simulink model "duocopter simulink model"  (R2020b)
settings: Solver=ode45  StartTime=0.0  StopTime=60  MaxStep=0.1  RelTol=1e-3
model workspace (MAT data in the model file):
  center_rotor_distance = 0.1
  mass_drone = 0.661
  moment_inertia_drone = [0.0019  0  0.0001; 0  0.004  0; 0.0001  0  0.0021]
  thrust_per_motor = 8.6328
libraries: simulink x6, pid_lib x3, shared6dof x1, robotcorelib x1, simulink_extras x1, sharedtransform x1, uavutilslib x1
settings Model: PacingRate=3  Creator=thega  LastModifiedBy=thega
settings DataIOCC: ReturnWorkspaceOutputsName=tp49ac784a_13d7_45a6_aa80_7f0641734b4f

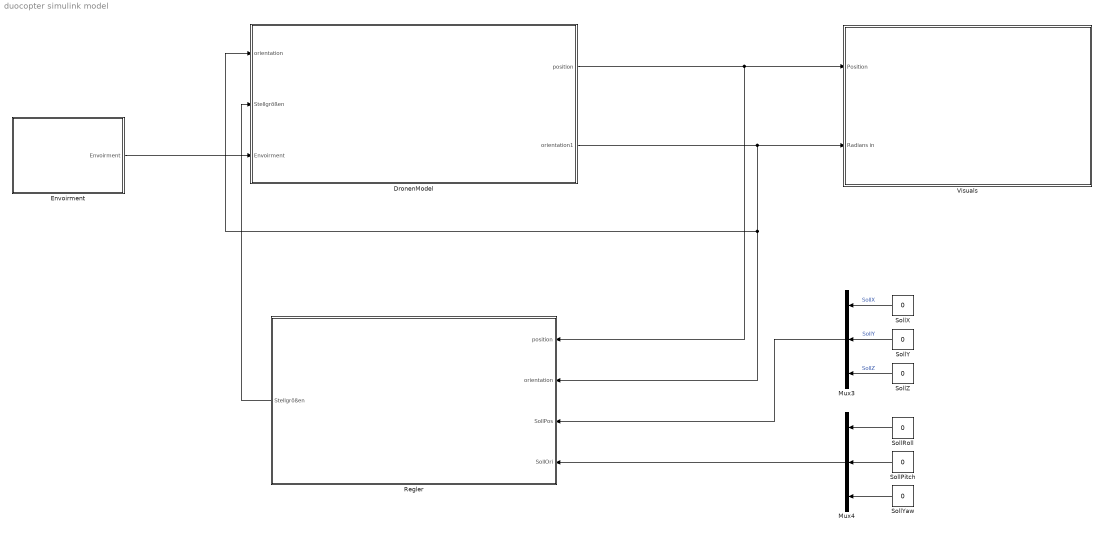
== system duocopter simulink model ==
  DronenModel : Subsystem
  Envoirment : Subsystem
  Mux3 : Mux  Inputs=3
  Mux4 : Mux  Inputs=3
  Regler : Subsystem
  SollPitch : Constant  Value=0
  SollRoll : Constant  Value=0
  SollX : Constant  Value=0
  SollY : Constant  Value=0
  SollYaw : Constant  Value=0
  SollZ : Constant  Value=0
  Visuals : Subsystem
  wires:
  SollX/1 -> Mux3/1  "SollX"
  SollY/1 -> Mux3/2  "SollY"
  SollZ/1 -> Mux3/3  "SollZ"
  SollYaw/1 -> Mux4/3
  SollPitch/1 -> Mux4/2
  SollRoll/1 -> Mux4/1
  Mux3/1 -> Regler/3(SollPos)
  Mux4/1 -> Regler/4(SollOri)
  DronenModel/1(position) -> Regler/1(position), Visuals/1(Position)
  DronenModel/2(orientation1) -> Visuals/2(Radians in), DronenModel/1(orientation), Regler/2(orientation)
  Regler/1(Stellgrößen) -> DronenModel/2(Stellgrößen)
  Envoirment/1(Envoirment) -> DronenModel/3(Envoirment)

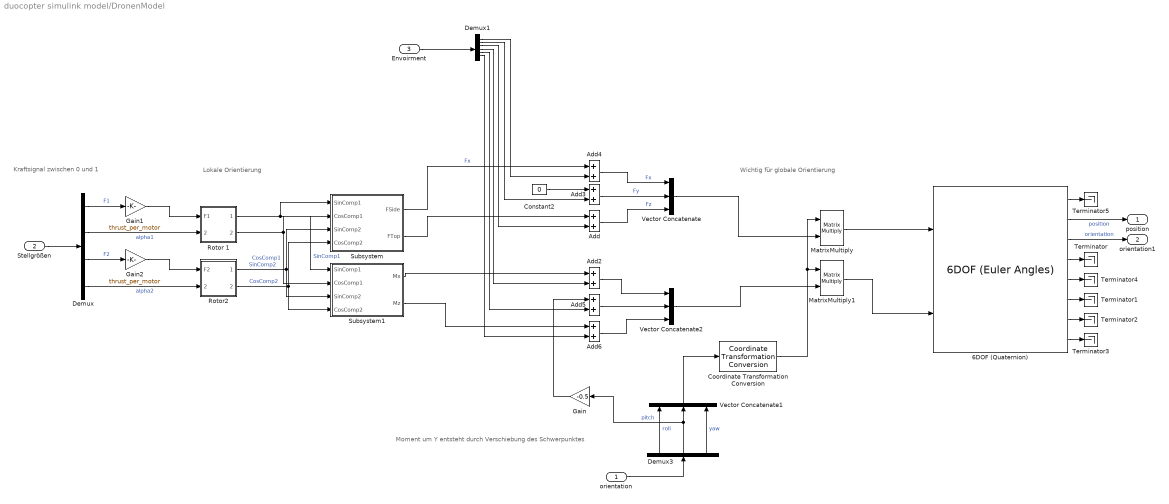
== system duocopter simulink model/DronenModel ==
  note: Kraftsignal zwischen 0 und 1
  note: Moment um Y entsteht durch Verschiebung des Schwerpunktes
  note: Lokale Orientierung
  note: Wichtig für globale Orientierung
  orientation : Inport
  Stellgrößen : Inport  Port=2
  Envoirment : Inport  Port=3
  6DOF (Quaternion) : shared6dof/6DOF (Euler Angles)  units=Metric (MKS)  mtype=Fixed  rep=Quaternion  xme_0=[0 0 0]  Vm_0=[0 0 0]  eul_0=[0 0 0]  pm_0=[0 0 0]  mass_0=mass_drone  mass_e=0.5  mass_f=2.0  inertia=moment_inertia_drone  inertia_e=eye(3)  inertia_f=2*eye(3)  k_quat=1.0  vre_flag=on  abi_flag=off  aMode=0  xme_statename=''  Vm_statename=''  eul_statename=''  quat_statename=''  pm_statename=''  mass_statename=''
      settings: SourceProductBaseCode=AE,PW,MT,UV,VE,VP
  Add{,2..6} (6 alike) : Sum
  Constant2 : Constant  Value=0
  Coordinate Transformation Conversion : robotcorelib/Coordinate Transformation Conversion  InputRepresentation=Euler Angles  InputEulerSequence=XYZ  ShowTrVecInputPort=on  OutputRepresentation=Rotation Matrix  OutputEulerSequence=ZYX  ShowTrVecOutputPort=on  SimulateUsing=Interpreted execution
      settings: SourceProductBaseCode=NV,RO,RR,UV
  Demux : Demux
  Demux1 : Demux  Outputs=6
  Demux3 : Demux  Outputs=3
  Gain : Gain  Gain=-0.5
  Gain1 : Gain  Gain=thrust_per_motor
  Gain2 : Gain  Gain=thrust_per_motor
  MatrixMultiply : Product  Multiplication=Matrix(*)
  MatrixMultiply1 : Product  Multiplication=Matrix(*)
  Rotor 1 : Subsystem
  Rotor2 : Subsystem
  Subsystem : Subsystem
  Subsystem1 : Subsystem
  Terminator{,1..5} (6 alike) : Terminator
  Vector Concatenate : Concatenate  NumInputs=3
  Vector Concatenate1 : Concatenate  NumInputs=3
  Vector Concatenate2 : Concatenate  NumInputs=3
  position : Outport
  orientation1 : Outport  Port=2
  wires:
  Add/1 -> Vector Concatenate/3  "Fz"
  6DOF (Quaternion)/8 -> Terminator3/1
  Demux3/3 -> Vector Concatenate1/3  "yaw"
  6DOF (Quaternion)/3 -> orientation1/1  "orientation"
  Rotor 1/2(Out2) -> Subsystem1/2(CosComp1), Subsystem/2(CosComp1)  "CosComp1"
  Rotor 1/1(Out1) -> Subsystem/1(SinComp1), Subsystem1/1(SinComp1)  "SinComp1"
  Subsystem/1(FSide) -> Add4/1  "Fx"
  Demux/1 -> Gain1/1  "F1"
  Subsystem1/1(Mx) -> Add2/1
  orientation/1 -> Demux3/1
  Rotor2/2(Out2) -> Subsystem1/4(CosComp2), Subsystem/4(CosComp2)  "CosComp2"
  Subsystem/2(FTop) -> Add/1
  Demux/2 -> Rotor 1/2(alpha1)  "alpha1"
  Demux3/1 -> Vector Concatenate1/1  "roll"
  Demux/4 -> Rotor2/2(alpha2)  "alpha2"
  6DOF (Quaternion)/7 -> Terminator2/1
  Rotor2/1(Out1) -> Subsystem1/3(SinComp2), Subsystem/3(SinComp2)  "SinComp2"
  Demux3/2 -> Gain/1, Vector Concatenate1/2  "pitch"
  6DOF (Quaternion)/2 -> position/1  "position"
  MatrixMultiply/1 -> 6DOF (Quaternion)/1
  6DOF (Quaternion)/4 -> Terminator/1
  Demux/3 -> Gain2/1  "F2"
  6DOF (Quaternion)/6 -> Terminator1/1
  6DOF (Quaternion)/1 -> Terminator5/1
  6DOF (Quaternion)/5 -> Terminator4/1
  Add3/1 -> Vector Concatenate/2  "Fy"
  Vector Concatenate/1 -> MatrixMultiply/2
  Vector Concatenate1/1 -> Coordinate Transformation Conversion/1
  Coordinate Transformation Conversion/1 -> MatrixMultiply/1, MatrixMultiply1/1
  Add2/1 -> Vector Concatenate2/1
  Add5/1 -> Vector Concatenate2/2
  Subsystem1/2(Mz) -> Add6/1
  Vector Concatenate2/1 -> MatrixMultiply1/2
  MatrixMultiply1/1 -> 6DOF (Quaternion)/2
  Add4/1 -> Vector Concatenate/1  "Fx"
  Demux1/2 -> Add3/2
  Demux1/1 -> Add4/2
  Demux1/3 -> Add/2
  Envoirment/1 -> Demux1/1
  Gain/1 -> Add5/1
  Add6/1 -> Vector Concatenate2/3
  Demux1/4 -> Add2/2
  Demux1/5 -> Add5/2
  Demux1/6 -> Add6/2
  Stellgrößen/1 -> Demux/1
  Constant2/1 -> Add3/1
  Gain1/1 -> Rotor 1/1(F1)
  Gain2/1 -> Rotor2/1(F2)

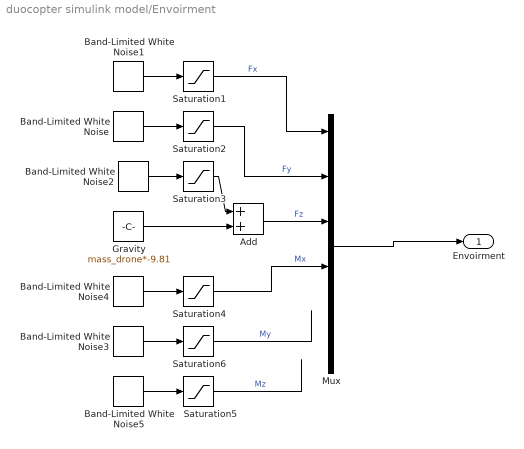
== system duocopter simulink model/Envoirment ==
  Add : Sum
  Band-Limited White Noise : simulink/Sources/Band-Limited White Noise  Cov=[0.1]  Ts=0.1  seed=[41]
  Band-Limited White Noise1 : simulink/Sources/Band-Limited White Noise  Cov=[0.1]  Ts=0.1  seed=[23222241]
  Band-Limited White Noise2 : simulink/Sources/Band-Limited White Noise  Cov=[0.1]  Ts=0.1  seed=[23341]
  Band-Limited White Noise3 : simulink/Sources/Band-Limited White Noise  Cov=[0.1]  Ts=0.1  seed=[67821]
  Band-Limited White Noise4 : simulink/Sources/Band-Limited White Noise  Cov=[0.001]  Ts=0.1  seed=[23678]
  Band-Limited White Noise5 : simulink/Sources/Band-Limited White Noise  Cov=[0.1]  Ts=0.1  seed=[2330]
  Gravity : Constant  Value=mass_drone*-9.81
  Mux : Mux  Inputs=6
  Saturation{1..3,5..6} (5 alike) : Saturate  UpperLimit=0.1  LowerLimit=-.1
  Saturation4 : Saturate  UpperLimit=0.001  LowerLimit=-.0001
  Envoirment : Outport
  wires:
  Mux/1 -> Envoirment/1
  Add/1 -> Mux/3  "Fz"
  Gravity/1 -> Add/2
  Band-Limited White Noise2/1 -> Saturation3/1
  Band-Limited White Noise/1 -> Saturation2/1
  Band-Limited White Noise1/1 -> Saturation1/1
  Band-Limited White Noise4/1 -> Saturation4/1
  Band-Limited White Noise3/1 -> Saturation6/1
  Band-Limited White Noise5/1 -> Saturation5/1
  Saturation1/1 -> Mux/1  "Fx"
  Saturation2/1 -> Mux/2  "Fy"
  Saturation3/1 -> Add/1
  Saturation4/1 -> Mux/4  "Mx"
  Saturation6/1 -> ?  "My"
  Saturation5/1 -> ?  "Mz"

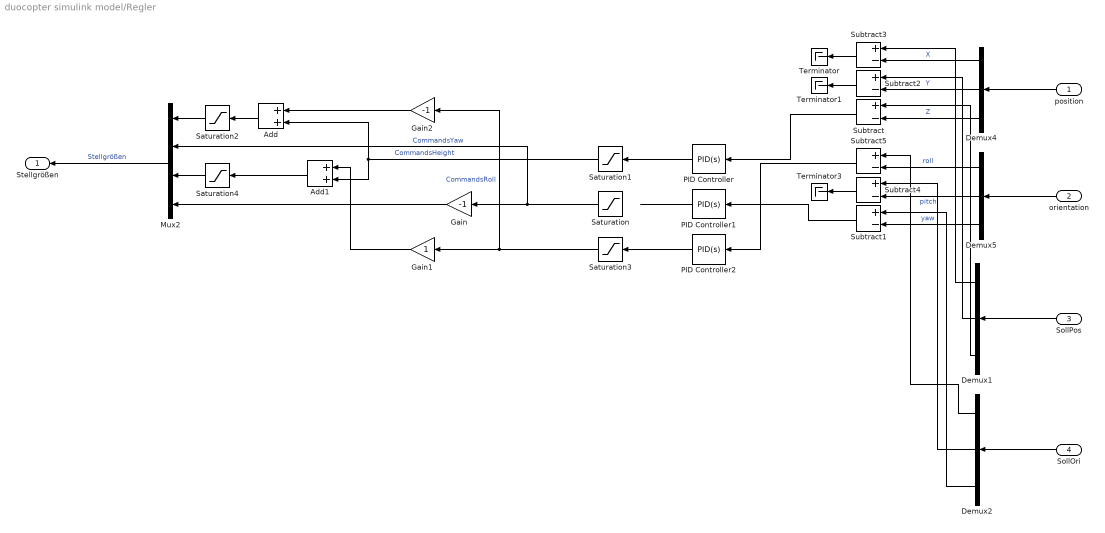
== system duocopter simulink model/Regler ==
  position : Inport
  orientation : Inport  Port=2
  SollPos : Inport  Port=3
  SollOri : Inport  Port=4
  Add : Sum
  Add1 : Sum
  Demux{1..2,4..5} (4 alike) : Demux  Outputs=3
  Gain : Gain  Gain=-1
  Gain1 : Gain
  Gain2 : Gain  Gain=-1
  Mux2 : Mux
  PID Controller : pid_lib/PID Controller  Controller=PID  Form=Parallel  TimeDomain=Continuous-time  UseExternalTs=off  SampleTime=-1  IntegratorMethod=Forward Euler  FilterMethod=Forward Euler  ControllerParametersSource=internal  P=0.0188303154649847  I=0.00247755067319415  D=0.0356353845754746  UseFilter=on  N=114.28279760416  TunerSelectOption=Transfer Function Based (PID Tuner App)  InitialConditionSource=internal  InitialConditionForIntegrator=0  InitialConditionForFilter=0  DifferentiatorICPrevScaledInput=0  ExternalReset=none  TrackingMode=off  Kt=1  LimitOutput=off  SatLimitsSource=internal  UpperSaturationLimit=inf  LowerSaturationLimit=-inf  LinearizeAsGain=on  AntiWindupMode=none  Kb=1  POutMin=[]  POutMax=[]  IOutMin=[]  IOutMax=[]  DOutMin=[]  DOutMax=[]  NOutMin=[]  NOutMax=[]  SumOutMin=[]  SumOutMax=[]  SaturationOutMin=[]  SaturationOutMax=[]  PParamMin=[]  PParamMax=[]  IParamMin=[]  IParamMax=[]  DParamMin=[]  DParamMax=[]  NParamMin=[]  NParamMax=[]  KbParamMin=[]  KbParamMax=[]  KtParamMin=[]  KtParamMax=[]  KbOutMin=[]  KbOutMax=[]  KtOutMin=[]  KtOutMax=[]  IntegratorOutMin=[]  IntegratorOutMax=[]  FilterOutMin=[]  FilterOutMax=[]  SumI1OutMin=[]  SumI1OutMax=[]  SumI2OutMin=[]  SumI2OutMax=[]  SumI3OutMin=[]  SumI3OutMax=[]  SumI4OutMin=[]  SumI4OutMax=[]  SumDOutMin=[]  SumDOutMax=[]  DifferentiatorOutMin=[]  DifferentiatorOutMax=[]  FilterDiffOutCoefMin=[]  FilterDiffOutCoefMax=[]  ReciprocalOutMin=[]  ReciprocalOutMax=[]  SumDenOutMin=[]  SumDenOutMax=[]  SumNumOutMin=[]  SumNumOutMax=[]  DivideOutMin=[]  DivideOutMax=[]  UdiffTsProdOutMin=[]  UdiffTsProdOutMax=[]  NTsProdOutMin=[]  NTsProdOutMax=[]  UintegralTsProdOutMin=[]  UintegralTsProdOutMax=[]  UngainTsProdOutMin=[]  UngainTsProdOutMax=[]  IntegratorContinuousStateAttributes=''  IntegratorStateMustResolveToSignalObject=off  IntegratorRTWStateStorageClass=Auto  FilterContinuousStateAttributes=''  FilterStateMustResolveToSignalObject=off  FilterRTWStateStorageClass=Auto  ParallelPVariant=InternalParameters  IdealPVariant=Disabled  IVariant=InternalParameters  DVariant=InternalParameters  IntegratorVariant=Continuous  SatVariant=Disabled  AWVariant=Passthrough  PCopyVariant=Disabled  TRVariant=Disabled  FdbkBlocksVariant=Forward  IdealPFdbkVariant=Disabled  SatFdbkVariant=Disabled  DerivativeFilterVariant=ContFilter  NVariant=InternalParameters  NCopyVariant=Disabled  FilterICVariant=InternalICsFilter  IntegratorICVariant=InternalICs  ExternalResetVariant=Disabled  TRSumVariant=Passthrough  SumFdbkVariant=Disabled  SumVariant=Sum_PID  TsampFilterVariant=InternalTs  TsampNgainVariant=Passthrough  TsampIntegralVariant=Passthrough  ExternalSaturationOutDataTypeStr=Inherit: Same as second input
  PID Controller1 : pid_lib/PID Controller  Controller=PID  Form=Parallel  TimeDomain=Continuous-time  UseExternalTs=off  SampleTime=-1  IntegratorMethod=Forward Euler  FilterMethod=Forward Euler  ControllerParametersSource=internal  P=0  I=-1  D=0  UseFilter=on  N=100  TunerSelectOption=Transfer Function Based (PID Tuner App)  InitialConditionSource=internal  InitialConditionForIntegrator=0  InitialConditionForFilter=0  DifferentiatorICPrevScaledInput=0  ExternalReset=none  TrackingMode=off  Kt=1  LimitOutput=off  SatLimitsSource=internal  UpperSaturationLimit=inf  LowerSaturationLimit=-inf  LinearizeAsGain=on  AntiWindupMode=none  Kb=1  POutMin=[]  POutMax=[]  IOutMin=[]  IOutMax=[]  DOutMin=[]  DOutMax=[]  NOutMin=[]  NOutMax=[]  SumOutMin=[]  SumOutMax=[]  SaturationOutMin=[]  SaturationOutMax=[]  PParamMin=[]  PParamMax=[]  IParamMin=[]  IParamMax=[]  DParamMin=[]  DParamMax=[]  NParamMin=[]  NParamMax=[]  KbParamMin=[]  KbParamMax=[]  KtParamMin=[]  KtParamMax=[]  KbOutMin=[]  KbOutMax=[]  KtOutMin=[]  KtOutMax=[]  IntegratorOutMin=[]  IntegratorOutMax=[]  FilterOutMin=[]  FilterOutMax=[]  SumI1OutMin=[]  SumI1OutMax=[]  SumI2OutMin=[]  SumI2OutMax=[]  SumI3OutMin=[]  SumI3OutMax=[]  SumI4OutMin=[]  SumI4OutMax=[]  SumDOutMin=[]  SumDOutMax=[]  DifferentiatorOutMin=[]  DifferentiatorOutMax=[]  FilterDiffOutCoefMin=[]  FilterDiffOutCoefMax=[]  ReciprocalOutMin=[]  ReciprocalOutMax=[]  SumDenOutMin=[]  SumDenOutMax=[]  SumNumOutMin=[]  SumNumOutMax=[]  DivideOutMin=[]  DivideOutMax=[]  UdiffTsProdOutMin=[]  UdiffTsProdOutMax=[]  NTsProdOutMin=[]  NTsProdOutMax=[]  UintegralTsProdOutMin=[]  UintegralTsProdOutMax=[]  UngainTsProdOutMin=[]  UngainTsProdOutMax=[]  IntegratorContinuousStateAttributes=''  IntegratorStateMustResolveToSignalObject=off  IntegratorRTWStateStorageClass=Auto  FilterContinuousStateAttributes=''  FilterStateMustResolveToSignalObject=off  FilterRTWStateStorageClass=Auto  ParallelPVariant=InternalParameters  IdealPVariant=Disabled  IVariant=InternalParameters  DVariant=InternalParameters  IntegratorVariant=Continuous  SatVariant=Disabled  AWVariant=Passthrough  PCopyVariant=Disabled  TRVariant=Disabled  FdbkBlocksVariant=Forward  IdealPFdbkVariant=Disabled  SatFdbkVariant=Disabled  DerivativeFilterVariant=ContFilter  NVariant=InternalParameters  NCopyVariant=Disabled  FilterICVariant=InternalICsFilter  IntegratorICVariant=InternalICs  ExternalResetVariant=Disabled  TRSumVariant=Passthrough  SumFdbkVariant=Disabled  SumVariant=Sum_PID  TsampFilterVariant=InternalTs  TsampNgainVariant=Passthrough  TsampIntegralVariant=Passthrough  ExternalSaturationOutDataTypeStr=Inherit: Same as second input
  PID Controller2 : pid_lib/PID Controller  Controller=PID  Form=Parallel  TimeDomain=Continuous-time  UseExternalTs=off  SampleTime=-1  IntegratorMethod=Forward Euler  FilterMethod=Forward Euler  ControllerParametersSource=internal  P=0.000203819394205205  I=9.54175974883443e-06  D=0.00106906921632501  UseFilter=on  N=5.45397025421619  TunerSelectOption=Transfer Function Based (PID Tuner App)  InitialConditionSource=internal  InitialConditionForIntegrator=0  InitialConditionForFilter=0  DifferentiatorICPrevScaledInput=0  ExternalReset=none  TrackingMode=off  Kt=1  LimitOutput=off  SatLimitsSource=internal  UpperSaturationLimit=inf  LowerSaturationLimit=-inf  LinearizeAsGain=on  AntiWindupMode=none  Kb=1  POutMin=[]  POutMax=[]  IOutMin=[]  IOutMax=[]  DOutMin=[]  DOutMax=[]  NOutMin=[]  NOutMax=[]  SumOutMin=[]  SumOutMax=[]  SaturationOutMin=[]  SaturationOutMax=[]  PParamMin=[]  PParamMax=[]  IParamMin=[]  IParamMax=[]  DParamMin=[]  DParamMax=[]  NParamMin=[]  NParamMax=[]  KbParamMin=[]  KbParamMax=[]  KtParamMin=[]  KtParamMax=[]  KbOutMin=[]  KbOutMax=[]  KtOutMin=[]  KtOutMax=[]  IntegratorOutMin=[]  IntegratorOutMax=[]  FilterOutMin=[]  FilterOutMax=[]  SumI1OutMin=[]  SumI1OutMax=[]  SumI2OutMin=[]  SumI2OutMax=[]  SumI3OutMin=[]  SumI3OutMax=[]  SumI4OutMin=[]  SumI4OutMax=[]  SumDOutMin=[]  SumDOutMax=[]  DifferentiatorOutMin=[]  DifferentiatorOutMax=[]  FilterDiffOutCoefMin=[]  FilterDiffOutCoefMax=[]  ReciprocalOutMin=[]  ReciprocalOutMax=[]  SumDenOutMin=[]  SumDenOutMax=[]  SumNumOutMin=[]  SumNumOutMax=[]  DivideOutMin=[]  DivideOutMax=[]  UdiffTsProdOutMin=[]  UdiffTsProdOutMax=[]  NTsProdOutMin=[]  NTsProdOutMax=[]  UintegralTsProdOutMin=[]  UintegralTsProdOutMax=[]  UngainTsProdOutMin=[]  UngainTsProdOutMax=[]  IntegratorContinuousStateAttributes=''  IntegratorStateMustResolveToSignalObject=off  IntegratorRTWStateStorageClass=Auto  FilterContinuousStateAttributes=''  FilterStateMustResolveToSignalObject=off  FilterRTWStateStorageClass=Auto  ParallelPVariant=InternalParameters  IdealPVariant=Disabled  IVariant=InternalParameters  DVariant=InternalParameters  IntegratorVariant=Continuous  SatVariant=Disabled  AWVariant=Passthrough  PCopyVariant=Disabled  TRVariant=Disabled  FdbkBlocksVariant=Forward  IdealPFdbkVariant=Disabled  SatFdbkVariant=Disabled  DerivativeFilterVariant=ContFilter  NVariant=InternalParameters  NCopyVariant=Disabled  FilterICVariant=InternalICsFilter  IntegratorICVariant=InternalICs  ExternalResetVariant=Disabled  TRSumVariant=Passthrough  SumFdbkVariant=Disabled  SumVariant=Sum_PID  TsampFilterVariant=InternalTs  TsampNgainVariant=Passthrough  TsampIntegralVariant=Passthrough  ExternalSaturationOutDataTypeStr=Inherit: Same as second input
  Saturation : Saturate  UpperLimit=1  LowerLimit=-1
  Saturation1 : Saturate  UpperLimit=1  LowerLimit=0
  Saturation2 : Saturate  UpperLimit=1  LowerLimit=0
  Saturation3 : Saturate  LowerLimit=0
  Saturation4 : Saturate  UpperLimit=1  LowerLimit=0
  Subtract{,1..5} (6 alike) : Sum  Inputs=+-
  Terminator : Terminator
  Terminator1 : Terminator
  Terminator3 : Terminator
  Stellgrößen : Outport
  wires:
  Demux1/2 -> Subtract2/1
  Demux2/2 -> Subtract4/1
  Saturation1/1 -> Add1/2, Add/2  "CommandsHeight"
  Subtract/1 -> PID Controller/1
  SollOri/1 -> Demux2/1
  PID Controller/1 -> Saturation1/1
  Demux5/3 -> Subtract1/2  "yaw"
  Demux1/1 -> Subtract3/1
  Subtract3/1 -> Terminator/1
  Mux2/1 -> Stellgrößen/1  "Stellgrößen"
  Subtract1/1 -> PID Controller1/1
  Demux4/3 -> Subtract/2  "Z"
  Demux2/3 -> Subtract1/1
  Saturation/1 -> Gain/1, Mux2/2  "CommandsYaw"
  Demux2/1 -> Subtract5/1
  Gain/1 -> Mux2/4
  Demux5/1 -> Subtract5/2  "roll"
  Demux1/3 -> Subtract/1
  Demux5/2 -> Subtract4/2  "pitch"
  Demux4/2 -> Subtract2/2  "Y"
  Demux4/1 -> Subtract3/2  "X"
  Subtract2/1 -> Terminator1/1
  SollPos/1 -> Demux1/1
  orientation/1 -> Demux5/1
  position/1 -> Demux4/1
  Saturation3/1 -> Gain2/1, Gain1/1  "CommandsRoll"
  Gain1/1 -> Add1/1
  Add/1 -> Saturation2/1
  Add1/1 -> Saturation4/1
  Subtract4/1 -> Terminator3/1
  Gain2/1 -> Add/1
  PID Controller1/1 -> ?
  PID Controller2/1 -> Saturation3/1
  Subtract5/1 -> PID Controller2/1
  Saturation4/1 -> Mux2/3
  Saturation2/1 -> Mux2/1

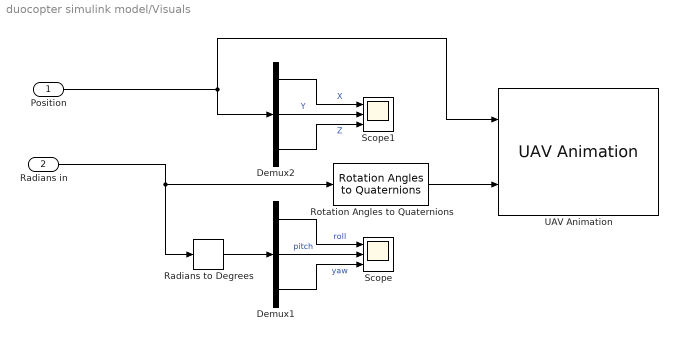
== system duocopter simulink model/Visuals ==
  Position : Inport
  Radians in : Inport  Port=2
  Demux1 : Demux  Outputs=3
  Demux2 : Demux  Outputs=3
  Radians to Degrees : simulink_extras/Transformations/Radians to Degrees
  Rotation Angles to Quaternions : sharedtransform/Rotation Angles to Quaternions  rotationOrder=XYZ  aMode=aMode
      settings: SourceProductBaseCode=AE,PW,MT,UV,VE,VP
  Scope : Scope  NumInputPorts=3
  Scope1 : Scope  NumInputPorts=3
  UAV Animation : uavutilslib/UAV Animation  UAVType=Multirotor  UAVSize=1  InertialZDirection=Up  SampleTime=-1
      settings: SourceProductBaseCode=UV
  wires:
  Radians to Degrees/1 -> Demux1/1
  Demux1/3 -> Scope/3  "yaw"
  Position/1 -> Demux2/1, UAV Animation/1
  Rotation Angles to Quaternions/1 -> UAV Animation/2
  Demux2/2 -> Scope1/2  "Y"
  Radians in/1 -> Radians to Degrees/1, Rotation Angles to Quaternions/1
  Demux1/2 -> Scope/2  "pitch"
  Demux1/1 -> Scope/1  "roll"
  Demux2/3 -> Scope1/3  "Z"
  Demux2/1 -> Scope1/1  "X"

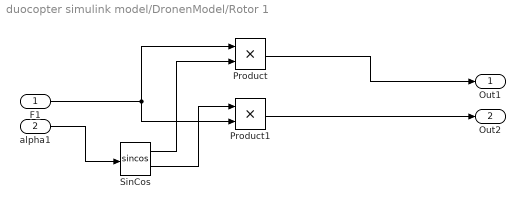
== system duocopter simulink model/DronenModel/Rotor 1 ==
  F1 : Inport
  alpha1 : Inport  Port=2
  Product : Product
  Product1 : Product
  SinCos : Trigonometry  Operator=sincos
  Out1 : Outport
  Out2 : Outport  Port=2
  wires:
  SinCos/2 -> Product1/1
  Product/1 -> Out1/1
  SinCos/1 -> Product/2
  F1/1 -> Product1/2, Product/1
  Product1/1 -> Out2/1
  alpha1/1 -> SinCos/1

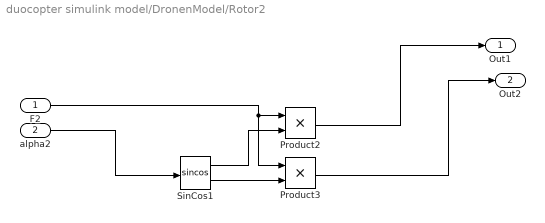
== system duocopter simulink model/DronenModel/Rotor2 ==
  F2 : Inport
  alpha2 : Inport  Port=2
  Product2 : Product
  Product3 : Product
  SinCos1 : Trigonometry  Operator=sincos
  Out1 : Outport
  Out2 : Outport  Port=2
  wires:
  SinCos1/1 -> Product2/2
  Product2/1 -> Out1/1
  SinCos1/2 -> Product3/2
  F2/1 -> Product2/1, Product3/1
  alpha2/1 -> SinCos1/1
  Product3/1 -> Out2/1

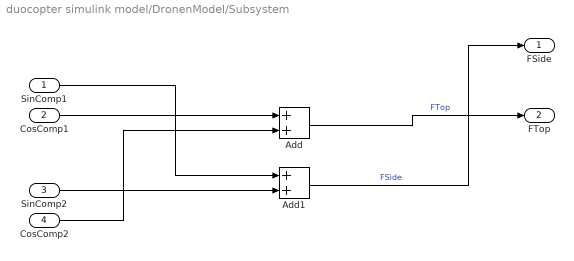
== system duocopter simulink model/DronenModel/Subsystem ==
  SinComp1 : Inport
  CosComp1 : Inport  Port=2
  SinComp2 : Inport  Port=3
  CosComp2 : Inport  Port=4
  Add : Sum
  Add1 : Sum
  FSide : Outport
  FTop : Outport  Port=2
  wires:
  Add1/1 -> FSide/1  "FSide"
  CosComp1/1 -> Add/1
  CosComp2/1 -> Add/2
  SinComp2/1 -> Add1/2
  Add/1 -> FTop/1  "FTop"
  SinComp1/1 -> Add1/1

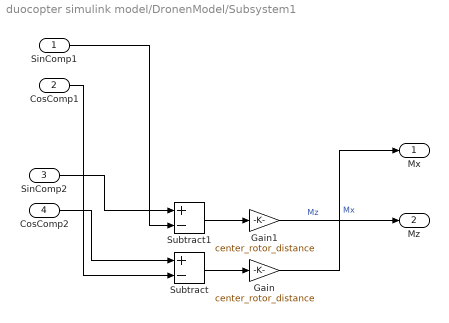
== system duocopter simulink model/DronenModel/Subsystem1 ==
  SinComp1 : Inport
  CosComp1 : Inport  Port=2
  SinComp2 : Inport  Port=3
  CosComp2 : Inport  Port=4
  Gain : Gain  Gain=center_rotor_distance
  Gain1 : Gain  Gain=center_rotor_distance
  Subtract : Sum  Inputs=+-
  Subtract1 : Sum  Inputs=+-
  Mx : Outport
  Mz : Outport  Port=2
  wires:
  Subtract1/1 -> Gain1/1
  CosComp1/1 -> Subtract/2
  Subtract/1 -> Gain/1
  Gain/1 -> Mx/1  "Mx"
  SinComp1/1 -> Subtract1/2
  Gain1/1 -> Mz/1  "Mz"
  CosComp2/1 -> Subtract/1
  SinComp2/1 -> Subtract1/1
